simulink model "linear_flight_controller_payload"  (R2020a)
settings: Solver=FixedStepAuto  StartTime=0.0  StopTime=50  FixedStep=0.005  RelTol=1e-3
InitFcn:
  | flight_controller_payload_setup % Script to setup workspace
values from neighbouring files (symbols this model uses):
  C_Dx = 0.2    [PID_design_setup.m]    (also in flight_controller_payload_setup.m)
  C_Dz = 0.2    [PID_design_setup.m]    (also in flight_controller_payload_setup.m)
  C_px = 0.05    [flight_controller_payload_setup.m]
  C_pz = 0.05    [flight_controller_payload_setup.m]
  cbeta = 0.05    [flight_controller_payload_setup.m]
  dtheta_sp_max = 120*pi/180    (= 2.09439510239)    [flight_controller_payload_setup.m]
  dtheta_sp_min = -120*pi/180    (= -2.09439510239)    [flight_controller_payload_setup.m]
  dx_sp_max = 12    [flight_controller_payload_setup.m]
  dx_sp_min = -12    [flight_controller_payload_setup.m]
  dz_sp_max = 12    [flight_controller_payload_setup.m]
  dz_sp_min = -12    [flight_controller_payload_setup.m]
  g = -9.81    [PID_design_setup.m]    (also in flight_controller_payload_setup.m)
  I_yy = 0.235    [PID_design_setup.m]    (also in flight_controller_payload_setup.m)
  ki_dtheta = kp_dtheta*z_c    (= 0.1)    [PID_design_setup.m]
  kp_dtheta = 10^(K_dB/20)    [PID_design_setup.m]
  l = 1    [flight_controller_payload_setup.m]
  M = 4.5    [PID_design_setup.m]    (also in flight_controller_payload_setup.m)
  m = 2    [flight_controller_payload_setup.m]
  MM = [-1, 1 ... (first row only)    [flight_controller_payload_setup.m]    (also in flight_controller_setup.m = [-1/sqrt(2), -1)
  N_dtheta = Inf    (= inf)    [flight_controller_payload_setup.m]
  N_dx = 5*2*pi    (= 31.4159265359)    [flight_controller_payload_setup.m]
  N_dz = 5*2*pi    (= 31.4159265359)    [flight_controller_payload_setup.m]
  r = 0.49*1/sqrt(2)    [PID_design_setup.m]    (also in flight_controller_payload_setup.m)
  rho = 1.225    [PID_design_setup.m]    (also in flight_controller_payload_setup.m)
  sigma = 0    [flight_controller_payload_setup.m]
  tau = 0.07    [PID_design_setup.m]    (also in flight_controller_payload_setup.m)
  theta_sp_max = 30*pi/180    (= 0.523598775598)    [flight_controller_payload_setup.m]
  theta_sp_min = -30*pi/180    (= -0.523598775598)    [flight_controller_payload_setup.m]
  Ts_excite = 0    [flight_controller_payload_setup.m]
  Ts_mpc = 0.03    [flight_controller_payload_setup.m]
  u0 = -0.5*M*g*[1; 1]    [flight_controller_payload_setup.m]
  var_excite = 0    [flight_controller_payload_setup.m]
  x0 = zeros(nx,1)    [flight_controller_payload_setup.m]    (also in flight_controller_setup.m = zeros(6,1))
  x0_no_load = zeros(6,1)    [flight_controller_payload_setup.m]
undefined symbols (not defined in the file or in its folder): A_lin, B_lin, kd_dtheta, kd_dx, kd_dz, ki_dx, ki_dz, kp_dx, kp_dz, kp_theta, kp_x, kp_z
libraries: simulink x26, dspstat3 x8, mpclib x2
(part 2 of 3)

== system linear_flight_controller_payload/PID controllers WITHOUT payload/Angular rate controller1 ==
  note: PID to use auto tuning from simulink
  dtheta_sp : Inport
  X : Inport  Port=2
  Demux1 : Demux  Outputs=6
  Derivative : Derivative
  Gain : Gain  Gain=kd_dtheta
  I : Gain  Gain=ki_dtheta
  Integrator Limited : Integrator  LimitOutput=on  UpperSaturationLimit=10  LowerSaturationLimit=-10
  Low Pass Filter : TransferFcn  Denominator=[1/N_dtheta, 1]
  P : Gain  Gain=kp_dtheta
  PID Omega Controller : simulink/Continuous/PID Controller  Commented=on  Controller=PID  Form=Parallel  TimeDomain=Continuous-time  UseExternalTs=off  SampleTime=-1  IntegratorMethod=Forward Euler  FilterMethod=Forward Euler  ControllerParametersSource=internal  P=kp_dtheta  I=ki_dtheta  D=kd_dtheta  UseFilter=on  N=N_dtheta  TunerSelectOption=Transfer Function Based (PID Tuner App)  InitialConditionSource=internal  InitialConditionForIntegrator=0  InitialConditionForFilter=0  DifferentiatorICPrevScaledInput=0  ExternalReset=none  TrackingMode=off  Kt=1  LimitOutput=off  UpperSaturationLimit=inf  LowerSaturationLimit=-inf  LinearizeAsGain=on  AntiWindupMode=none  Kb=1  POutMin=[]  POutMax=[]  IOutMin=[]  IOutMax=[]  DOutMin=[]  DOutMax=[]  NOutMin=[]  NOutMax=[]  SumOutMin=[]  SumOutMax=[]  SaturationOutMin=[]  SaturationOutMax=[]  PParamMin=[]  PParamMax=[]  IParamMin=[]  IParamMax=[]  DParamMin=[]  DParamMax=[]  NParamMin=[]  NParamMax=[]  KbParamMin=[]  KbParamMax=[]  KtParamMin=[]  KtParamMax=[]  KbOutMin=[]  KbOutMax=[]  KtOutMin=[]  KtOutMax=[]  IntegratorOutMin=[]  IntegratorOutMax=[]  FilterOutMin=[]  FilterOutMax=[]  SumI1OutMin=[]  SumI1OutMax=[]  SumI2OutMin=[]  SumI2OutMax=[]  SumI3OutMin=[]  SumI3OutMax=[]  SumI4OutMin=[]  SumI4OutMax=[]  SumDOutMin=[]  SumDOutMax=[]  DifferentiatorOutMin=[]  DifferentiatorOutMax=[]  FilterDiffOutCoefMin=[]  FilterDiffOutCoefMax=[]  ReciprocalOutMin=[]  ReciprocalOutMax=[]  SumDenOutMin=[]  SumDenOutMax=[]  SumNumOutMin=[]  SumNumOutMax=[]  DivideOutMin=[]  DivideOutMax=[]  UdiffTsProdOutMin=[]  UdiffTsProdOutMax=[]  NTsProdOutMin=[]  NTsProdOutMax=[]  UintegralTsProdOutMin=[]  UintegralTsProdOutMax=[]  UngainTsProdOutMin=[]  UngainTsProdOutMax=[]  IntegratorContinuousStateAttributes=''  IntegratorStateMustResolveToSignalObject=off  IntegratorRTWStateStorageClass=Auto  FilterContinuousStateAttributes=''  FilterStateMustResolveToSignalObject=off  FilterRTWStateStorageClass=Auto  ParallelPVariant=InternalParameters  IdealPVariant=Disabled  IVariant=InternalParameters  DVariant=InternalParameters  IntegratorVariant=Continuous  SatVariant=Disabled  AWVariant=Passthrough  PCopyVariant=Disabled  TRVariant=Disabled  FdbkBlocksVariant=Forward  IdealPFdbkVariant=Disabled  SatFdbkVariant=Disabled  DerivativeFilterVariant=ContFilter  NVariant=InternalParameters  NCopyVariant=Disabled  FilterICVariant=InternalICsFilter  IntegratorICVariant=InternalICs  ExternalResetVariant=Disabled  TRSumVariant=Passthrough  SumFdbkVariant=Disabled  SumVariant=Sum_PID  TsampFilterVariant=InternalTs  TsampNgainVariant=Passthrough  TsampIntegralVariant=Passthrough
  Sum : Sum  Inputs=|+-
  Sum1 : Sum  Inputs=++-
  Sum2 : Sum  Inputs=++|
  delta_E : Outport
  wires:
  dtheta_sp/1 -> Sum/1
  Sum/1 -> P/1, Integrator Limited/1, PID Omega Controller/1
  Integrator Limited/1 -> I/1
  Derivative/1 -> Gain/1
  I/1 -> Sum1/2
  P/1 -> Sum1/1
  Gain/1 -> Sum1/3
  Sum1/1 -> Sum2/2
  Sum2/1 -> delta_E/1
  PID Omega Controller/1 -> Sum2/1
  Low Pass Filter/1 -> Derivative/1
  X/1 -> Demux1/1
  Demux1/6 -> Low Pass Filter/1, Sum/2  "dtheta"

== system linear_flight_controller_payload/PID controllers WITHOUT payload/Motor Mixing Algorithm1 ==
  delta_E : Inport
  delta_T : Inport  Port=2
  Mixing Matrix : Gain  Gain=MM  Multiplication=Matrix(K*u)
  Mux : Mux  Inputs=2
  Signal Specification : SignalSpecification  Dimensions=[2, 1]
  u : Outport  LockScale=on
  wires:
  delta_T/1 -> Mux/2
  delta_E/1 -> Mux/1
  Mixing Matrix/1 -> u/1
  Mux/1 -> Signal Specification/1
  Signal Specification/1 -> Mixing Matrix/1

== system linear_flight_controller_payload/PID controllers WITHOUT payload/Plant WITHOUT payload ==
  u : Inport  PortDimensions=[2, 1]
  Integrator : Integrator  InitialCondition=x0_no_load
  MATLAB Function1 : MATLAB Function  TreatAsAtomicUnit=on
  Motors : Subsystem
  Signal Specification : SignalSpecification  Dimensions=2
  parameters : Subsystem
  x : Outport
  wires:
  Motors/1(T) -> Signal Specification/1
  Signal Specification/1 -> MATLAB Function1/2(u)
  MATLAB Function1/1(dx) -> Integrator/1
  u/1 -> Motors/1(T_r)
  parameters/1(parameters) -> MATLAB Function1/3(params)
  Integrator/1 -> x/1, MATLAB Function1/1(x)

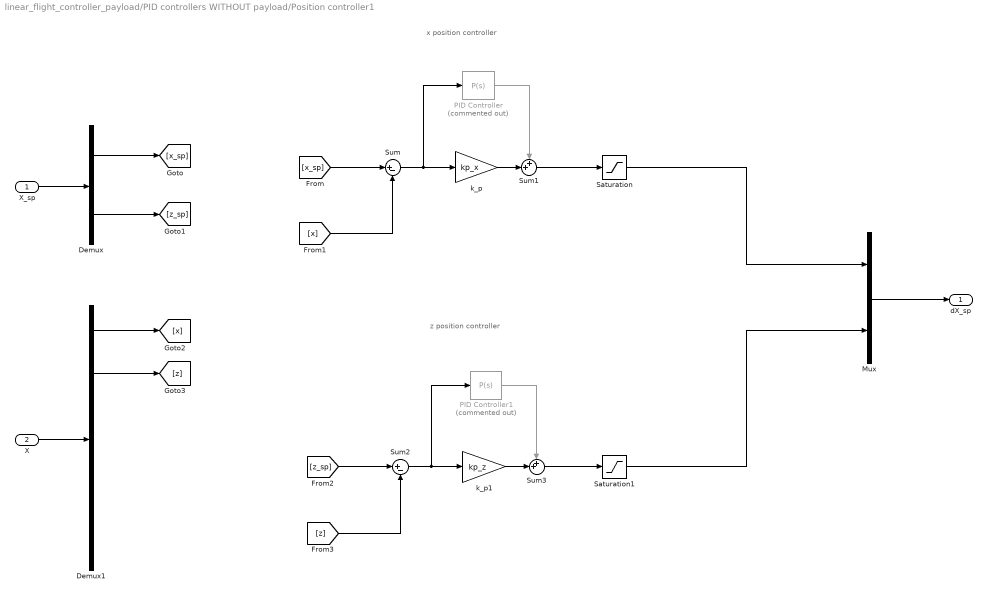
== system linear_flight_controller_payload/PID controllers WITHOUT payload/Position controller1 ==
  note: x position controller
  note: z position controller
  X_sp : Inport
  X : Inport  Port=2
  Demux : Demux  Outputs=2
  Demux1 : Demux  Outputs=6
  Mux : Mux  Inputs=2
  PID Controller : simulink/Continuous/PID Controller  Commented=on  Controller=P  Form=Parallel  TimeDomain=Continuous-time  UseExternalTs=off  SampleTime=-1  IntegratorMethod=Forward Euler  FilterMethod=Forward Euler  ControllerParametersSource=internal  P=20  I=1  D=0  UseFilter=on  N=100  TunerSelectOption=Transfer Function Based (PID Tuner App)  InitialConditionSource=internal  InitialConditionForIntegrator=0  InitialConditionForFilter=0  DifferentiatorICPrevScaledInput=0  ExternalReset=none  TrackingMode=off  Kt=1  LimitOutput=off  UpperSaturationLimit=inf  LowerSaturationLimit=-inf  LinearizeAsGain=on  AntiWindupMode=none  Kb=1  POutMin=[]  POutMax=[]  IOutMin=[]  IOutMax=[]  DOutMin=[]  DOutMax=[]  NOutMin=[]  NOutMax=[]  SumOutMin=[]  SumOutMax=[]  SaturationOutMin=[]  SaturationOutMax=[]  PParamMin=[]  PParamMax=[]  IParamMin=[]  IParamMax=[]  DParamMin=[]  DParamMax=[]  NParamMin=[]  NParamMax=[]  KbParamMin=[]  KbParamMax=[]  KtParamMin=[]  KtParamMax=[]  KbOutMin=[]  KbOutMax=[]  KtOutMin=[]  KtOutMax=[]  IntegratorOutMin=[]  IntegratorOutMax=[]  FilterOutMin=[]  FilterOutMax=[]  SumI1OutMin=[]  SumI1OutMax=[]  SumI2OutMin=[]  SumI2OutMax=[]  SumI3OutMin=[]  SumI3OutMax=[]  SumI4OutMin=[]  SumI4OutMax=[]  SumDOutMin=[]  SumDOutMax=[]  DifferentiatorOutMin=[]  DifferentiatorOutMax=[]  FilterDiffOutCoefMin=[]  FilterDiffOutCoefMax=[]  ReciprocalOutMin=[]  ReciprocalOutMax=[]  SumDenOutMin=[]  SumDenOutMax=[]  SumNumOutMin=[]  SumNumOutMax=[]  DivideOutMin=[]  DivideOutMax=[]  UdiffTsProdOutMin=[]  UdiffTsProdOutMax=[]  NTsProdOutMin=[]  NTsProdOutMax=[]  UintegralTsProdOutMin=[]  UintegralTsProdOutMax=[]  UngainTsProdOutMin=[]  UngainTsProdOutMax=[]  IntegratorContinuousStateAttributes=''  IntegratorStateMustResolveToSignalObject=off  IntegratorRTWStateStorageClass=Auto  FilterContinuousStateAttributes=''  FilterStateMustResolveToSignalObject=off  FilterRTWStateStorageClass=Auto  ParallelPVariant=InternalParameters  IdealPVariant=Disabled  IVariant=Disabled  DVariant=Disabled  IntegratorVariant=Disabled  SatVariant=Disabled  AWVariant=Disabled  PCopyVariant=Disabled  TRVariant=Disabled  FdbkBlocksVariant=Forward  IdealPFdbkVariant=Disabled  SatFdbkVariant=Disabled  DerivativeFilterVariant=Disabled  NVariant=Disabled  NCopyVariant=Disabled_SignalSpec  FilterICVariant=Disabled  IntegratorICVariant=Disabled  ExternalResetVariant=Disabled  TRSumVariant=Passthrough  SumFdbkVariant=Disabled  SumVariant=Passthrough_P  TsampFilterVariant=InternalTs  TsampNgainVariant=Passthrough  TsampIntegralVariant=Disabled_SignalSpec
  PID Controller1 : simulink/Continuous/PID Controller  Commented=on  Controller=P  Form=Parallel  TimeDomain=Continuous-time  UseExternalTs=off  SampleTime=-1  IntegratorMethod=Forward Euler  FilterMethod=Forward Euler  ControllerParametersSource=internal  P=1  I=1  D=0  UseFilter=on  N=100  TunerSelectOption=Transfer Function Based (PID Tuner App)  InitialConditionSource=internal  InitialConditionForIntegrator=0  InitialConditionForFilter=0  DifferentiatorICPrevScaledInput=0  ExternalReset=none  TrackingMode=off  Kt=1  LimitOutput=off  UpperSaturationLimit=inf  LowerSaturationLimit=-inf  LinearizeAsGain=on  AntiWindupMode=none  Kb=1  POutMin=[]  POutMax=[]  IOutMin=[]  IOutMax=[]  DOutMin=[]  DOutMax=[]  NOutMin=[]  NOutMax=[]  SumOutMin=[]  SumOutMax=[]  SaturationOutMin=[]  SaturationOutMax=[]  PParamMin=[]  PParamMax=[]  IParamMin=[]  IParamMax=[]  DParamMin=[]  DParamMax=[]  NParamMin=[]  NParamMax=[]  KbParamMin=[]  KbParamMax=[]  KtParamMin=[]  KtParamMax=[]  KbOutMin=[]  KbOutMax=[]  KtOutMin=[]  KtOutMax=[]  IntegratorOutMin=[]  IntegratorOutMax=[]  FilterOutMin=[]  FilterOutMax=[]  SumI1OutMin=[]  SumI1OutMax=[]  SumI2OutMin=[]  SumI2OutMax=[]  SumI3OutMin=[]  SumI3OutMax=[]  SumI4OutMin=[]  SumI4OutMax=[]  SumDOutMin=[]  SumDOutMax=[]  DifferentiatorOutMin=[]  DifferentiatorOutMax=[]  FilterDiffOutCoefMin=[]  FilterDiffOutCoefMax=[]  ReciprocalOutMin=[]  ReciprocalOutMax=[]  SumDenOutMin=[]  SumDenOutMax=[]  SumNumOutMin=[]  SumNumOutMax=[]  DivideOutMin=[]  DivideOutMax=[]  UdiffTsProdOutMin=[]  UdiffTsProdOutMax=[]  NTsProdOutMin=[]  NTsProdOutMax=[]  UintegralTsProdOutMin=[]  UintegralTsProdOutMax=[]  UngainTsProdOutMin=[]  UngainTsProdOutMax=[]  IntegratorContinuousStateAttributes=''  IntegratorStateMustResolveToSignalObject=off  IntegratorRTWStateStorageClass=Auto  FilterContinuousStateAttributes=''  FilterStateMustResolveToSignalObject=off  FilterRTWStateStorageClass=Auto  ParallelPVariant=InternalParameters  IdealPVariant=Disabled  IVariant=Disabled  DVariant=Disabled  IntegratorVariant=Disabled  SatVariant=Disabled  AWVariant=Disabled  PCopyVariant=Disabled  TRVariant=Disabled  FdbkBlocksVariant=Forward  IdealPFdbkVariant=Disabled  SatFdbkVariant=Disabled  DerivativeFilterVariant=Disabled  NVariant=Disabled  NCopyVariant=Disabled_SignalSpec  FilterICVariant=Disabled  IntegratorICVariant=Disabled  ExternalResetVariant=Disabled  TRSumVariant=Passthrough  SumFdbkVariant=Disabled  SumVariant=Passthrough_P  TsampFilterVariant=InternalTs  TsampNgainVariant=Passthrough  TsampIntegralVariant=Disabled_SignalSpec
  Saturation : Saturate  UpperLimit=dx_sp_max  LowerLimit=dx_sp_min
  Saturation1 : Saturate  UpperLimit=dz_sp_max  LowerLimit=dz_sp_min
  Sum : Sum  Inputs=|+-
  Sum1 : Sum  Inputs=++|
  Sum2 : Sum  Inputs=|+-
  Sum3 : Sum  Inputs=++|
  k_p : Gain  Gain=kp_x
  k_p1 : Gain  Gain=kp_z
  dX_sp : Outport
  wires:
  Sum/1 -> PID Controller/1, k_p/1
  k_p/1 -> Sum1/2
  PID Controller/1 -> Sum1/1
  X_sp/1 -> Demux/1
  Demux/2 -> [z_sp]
  Demux/1 -> [x_sp]
  X/1 -> Demux1/1
  Demux1/1 -> [x]
  Demux1/2 -> [z]
  [x_sp] -> Sum/1
  [x] -> Sum/2
  Sum2/1 -> PID Controller1/1, k_p1/1
  [z] -> Sum2/2
  [z_sp] -> Sum2/1
  PID Controller1/1 -> Sum3/1
  k_p1/1 -> Sum3/2
  Mux/1 -> dX_sp/1
  Sum1/1 -> Saturation/1
  Sum3/1 -> Saturation1/1
  Saturation1/1 -> Mux/2
  Saturation/1 -> Mux/1

== system linear_flight_controller_payload/PID controllers WITHOUT payload/Subsystem1 ==
  X : Inport
  Demux : Demux  Outputs=6
  theta : Outport
  wires:
  X/1 -> Demux/1
  Demux/3 -> theta/1

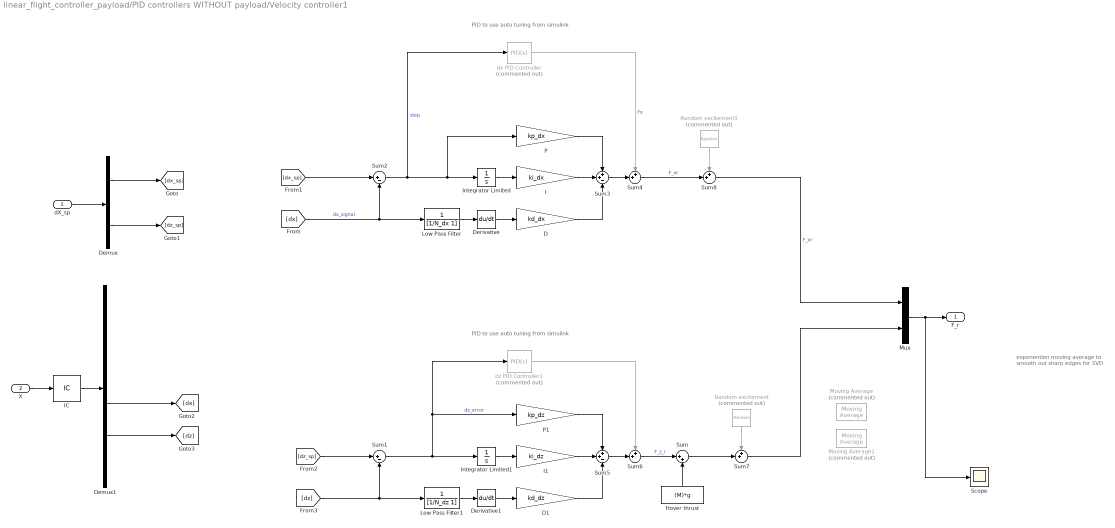
== system linear_flight_controller_payload/PID controllers WITHOUT payload/Velocity controller1 ==
  note: exponention moving average
      | to smooth out sharp edges for SVD
  note: PID to use auto tuning from simulink
  note: PID to use auto tuning from simulink
  dX_sp : Inport
  X : Inport  Port=2
  D : Gain  Gain=kd_dx
  D1 : Gain  Gain=kd_dz
  Demux : Demux  Outputs=2
  Demux1 : Demux  Outputs=6
  Derivative : Derivative
  Derivative1 : Derivative
  Hover thrust : Constant  Value=(M)*g
  I : Gain  Gain=ki_dx
  I1 : Gain  Gain=ki_dz
  IC : InitialCondition  Value=x0_no_load
  Integrator Limited : Integrator  LimitOutput=on  UpperSaturationLimit=10  LowerSaturationLimit=-10
  Integrator Limited1 : Integrator  LimitOutput=on  UpperSaturationLimit=10  LowerSaturationLimit=-10
  Low Pass Filter : TransferFcn  Denominator=[1/N_dx 1]
  Low Pass Filter1 : TransferFcn  Denominator=[1/N_dz 1]
  Moving Average : dspstat3/Moving Average  Commented=on  Method=Exponential weighting  ForgettingFactorPort=off  SpecifyWindowLength=on  WindowLength=4  ForgettingFactor=lambda  SimulateUsing=Code generation
  Moving Average1 : dspstat3/Moving Average  Commented=on  Method=Exponential weighting  ForgettingFactorPort=off  SpecifyWindowLength=on  WindowLength=4  ForgettingFactor=lambda  SimulateUsing=Code generation
  Mux : Mux  Inputs=2
  P : Gain  Gain=kp_dx
  P1 : Gain  Gain=kp_dz
  Random excitement : RandomNumber  Commented=on  Variance=var_excite  SampleTime=Ts_excite
  Random excitement1 : RandomNumber  Commented=on  Variance=var_excite  Seed=1  SampleTime=Ts_excite
  Scope : Scope
  Sum : Sum  Inputs=|++
  Sum1 : Sum  Inputs=|+-
  Sum2 : Sum  Inputs=|+-
  Sum3 : Sum  Inputs=++-
  Sum{4,6..8} (4 alike) : Sum  Inputs=++|
  Sum5 : Sum  Inputs=++-
  dx PID Controller : simulink/Continuous/PID Controller  Commented=on  Controller=PID  Form=Parallel  TimeDomain=Continuous-time  UseExternalTs=off  SampleTime=-1  IntegratorMethod=Forward Euler  FilterMethod=Forward Euler  ControllerParametersSource=internal  P=kp_dx  I=ki_dx  D=kd_dx  UseFilter=on  N=N_dx  TunerSelectOption=Transfer Function Based (PID Tuner App)  InitialConditionSource=internal  InitialConditionForIntegrator=0  InitialConditionForFilter=0  DifferentiatorICPrevScaledInput=0  ExternalReset=none  TrackingMode=off  Kt=1  LimitOutput=off  UpperSaturationLimit=inf  LowerSaturationLimit=-inf  LinearizeAsGain=on  AntiWindupMode=none  Kb=1  POutMin=[]  POutMax=[]  IOutMin=[]  IOutMax=[]  DOutMin=[]  DOutMax=[]  NOutMin=[]  NOutMax=[]  SumOutMin=[]  SumOutMax=[]  SaturationOutMin=[]  SaturationOutMax=[]  PParamMin=[]  PParamMax=[]  IParamMin=[]  IParamMax=[]  DParamMin=[]  DParamMax=[]  NParamMin=[]  NParamMax=[]  KbParamMin=[]  KbParamMax=[]  KtParamMin=[]  KtParamMax=[]  KbOutMin=[]  KbOutMax=[]  KtOutMin=[]  KtOutMax=[]  IntegratorOutMin=[]  IntegratorOutMax=[]  FilterOutMin=[]  FilterOutMax=[]  SumI1OutMin=[]  SumI1OutMax=[]  SumI2OutMin=[]  SumI2OutMax=[]  SumI3OutMin=[]  SumI3OutMax=[]  SumI4OutMin=[]  SumI4OutMax=[]  SumDOutMin=[]  SumDOutMax=[]  DifferentiatorOutMin=[]  DifferentiatorOutMax=[]  FilterDiffOutCoefMin=[]  FilterDiffOutCoefMax=[]  ReciprocalOutMin=[]  ReciprocalOutMax=[]  SumDenOutMin=[]  SumDenOutMax=[]  SumNumOutMin=[]  SumNumOutMax=[]  DivideOutMin=[]  DivideOutMax=[]  UdiffTsProdOutMin=[]  UdiffTsProdOutMax=[]  NTsProdOutMin=[]  NTsProdOutMax=[]  UintegralTsProdOutMin=[]  UintegralTsProdOutMax=[]  UngainTsProdOutMin=[]  UngainTsProdOutMax=[]  IntegratorContinuousStateAttributes=''  IntegratorStateMustResolveToSignalObject=off  IntegratorRTWStateStorageClass=Auto  FilterContinuousStateAttributes=''  FilterStateMustResolveToSignalObject=off  FilterRTWStateStorageClass=Auto  ParallelPVariant=InternalParameters  IdealPVariant=Disabled  IVariant=InternalParameters  DVariant=InternalParameters  IntegratorVariant=Continuous  SatVariant=Disabled  AWVariant=Passthrough  PCopyVariant=Disabled  TRVariant=Disabled  FdbkBlocksVariant=Forward  IdealPFdbkVariant=Disabled  SatFdbkVariant=Disabled  DerivativeFilterVariant=ContFilter  NVariant=InternalParameters  NCopyVariant=Disabled  FilterICVariant=InternalICsFilter  IntegratorICVariant=InternalICs  ExternalResetVariant=Disabled  TRSumVariant=Passthrough  SumFdbkVariant=Disabled  SumVariant=Sum_PID  TsampFilterVariant=InternalTs  TsampNgainVariant=Passthrough  TsampIntegralVariant=Passthrough
  dz PID Controller1 : simulink/Continuous/PID Controller  Commented=on  Controller=PID  Form=Parallel  TimeDomain=Continuous-time  UseExternalTs=off  SampleTime=-1  IntegratorMethod=Forward Euler  FilterMethod=Forward Euler  ControllerParametersSource=internal  P=kp_dz  I=ki_dz  D=kd_dz  UseFilter=on  N=N_dz  TunerSelectOption=Transfer Function Based (PID Tuner App)  InitialConditionSource=internal  InitialConditionForIntegrator=0  InitialConditionForFilter=0  DifferentiatorICPrevScaledInput=0  ExternalReset=none  TrackingMode=off  Kt=1  LimitOutput=off  UpperSaturationLimit=inf  LowerSaturationLimit=-inf  LinearizeAsGain=on  AntiWindupMode=none  Kb=1  POutMin=[]  POutMax=[]  IOutMin=[]  IOutMax=[]  DOutMin=[]  DOutMax=[]  NOutMin=[]  NOutMax=[]  SumOutMin=[]  SumOutMax=[]  SaturationOutMin=[]  SaturationOutMax=[]  PParamMin=[]  PParamMax=[]  IParamMin=[]  IParamMax=[]  DParamMin=[]  DParamMax=[]  NParamMin=[]  NParamMax=[]  KbParamMin=[]  KbParamMax=[]  KtParamMin=[]  KtParamMax=[]  KbOutMin=[]  KbOutMax=[]  KtOutMin=[]  KtOutMax=[]  IntegratorOutMin=[]  IntegratorOutMax=[]  FilterOutMin=[]  FilterOutMax=[]  SumI1OutMin=[]  SumI1OutMax=[]  SumI2OutMin=[]  SumI2OutMax=[]  SumI3OutMin=[]  SumI3OutMax=[]  SumI4OutMin=[]  SumI4OutMax=[]  SumDOutMin=[]  SumDOutMax=[]  DifferentiatorOutMin=[]  DifferentiatorOutMax=[]  FilterDiffOutCoefMin=[]  FilterDiffOutCoefMax=[]  ReciprocalOutMin=[]  ReciprocalOutMax=[]  SumDenOutMin=[]  SumDenOutMax=[]  SumNumOutMin=[]  SumNumOutMax=[]  DivideOutMin=[]  DivideOutMax=[]  UdiffTsProdOutMin=[]  UdiffTsProdOutMax=[]  NTsProdOutMin=[]  NTsProdOutMax=[]  UintegralTsProdOutMin=[]  UintegralTsProdOutMax=[]  UngainTsProdOutMin=[]  UngainTsProdOutMax=[]  IntegratorContinuousStateAttributes=''  IntegratorStateMustResolveToSignalObject=off  IntegratorRTWStateStorageClass=Auto  FilterContinuousStateAttributes=''  FilterStateMustResolveToSignalObject=off  FilterRTWStateStorageClass=Auto  ParallelPVariant=InternalParameters  IdealPVariant=Disabled  IVariant=InternalParameters  DVariant=InternalParameters  IntegratorVariant=Continuous  SatVariant=Disabled  AWVariant=Passthrough  PCopyVariant=Disabled  TRVariant=Disabled  FdbkBlocksVariant=Forward  IdealPFdbkVariant=Disabled  SatFdbkVariant=Disabled  DerivativeFilterVariant=ContFilter  NVariant=InternalParameters  NCopyVariant=Disabled  FilterICVariant=InternalICsFilter  IntegratorICVariant=InternalICs  ExternalResetVariant=Disabled  TRSumVariant=Passthrough  SumFdbkVariant=Disabled  SumVariant=Sum_PID  TsampFilterVariant=InternalTs  TsampNgainVariant=Passthrough  TsampIntegralVariant=Passthrough
  F_r : Outport
  wires:
  Derivative/1 -> D/1
  Sum3/1 -> Sum4/2
  Sum2/1 -> dx PID Controller/1, P/1, Integrator Limited/1  "step"
  I/1 -> Sum3/2
  Integrator Limited/1 -> I/1
  dx PID Controller/1 -> Sum4/1  "Fx"
  P/1 -> Sum3/1
  Low Pass Filter/1 -> Derivative/1
  D/1 -> Sum3/3
  P1/1 -> Sum5/1
  Integrator Limited1/1 -> I1/1
  dz PID Controller1/1 -> Sum6/1
  I1/1 -> Sum5/2
  Sum1/1 -> P1/1, dz PID Controller1/1, Integrator Limited1/1  "dz_error"
  Sum5/1 -> Sum6/2
  Low Pass Filter1/1 -> Derivative1/1
  Derivative1/1 -> D1/1
  D1/1 -> Sum5/3
  dX_sp/1 -> Demux/1
  [dx] -> Sum2/2, Low Pass Filter/1  "dx_signal"
  [dx_sp] -> Sum2/1
  Demux/1 -> [dx_sp]
  Demux/2 -> [dz_sp]
  [dz] -> Sum1/2, Low Pass Filter1/1
  [dz_sp] -> Sum1/1
  Demux1/4 -> [dx]
  Demux1/5 -> [dz]
  Sum6/1 -> Sum/1  "F_z_r"
  Hover thrust/1 -> Sum/2
  IC/1 -> Demux1/1
  X/1 -> IC/1
  Sum8/1 -> Mux/1  "F_xr"
  Sum7/1 -> Mux/2
  Mux/1 -> Scope/1, F_r/1
  Random excitement/1 -> Sum7/1
  Sum/1 -> Sum7/2
  Random excitement1/1 -> Sum8/1
  Sum4/1 -> Sum8/2  "F_xr"

== system linear_flight_controller_payload/PID controllers and Plant/Angle controller1 ==
  theta_sp : Inport
  X : Inport  Port=2
  Demux1 : Demux  Outputs=nx
  Gain : Gain  Gain=kp_theta
  PID Controller : simulink/Continuous/PID Controller  Commented=on  Controller=P  Form=Parallel  TimeDomain=Continuous-time  UseExternalTs=off  SampleTime=-1  IntegratorMethod=Forward Euler  FilterMethod=Forward Euler  ControllerParametersSource=internal  P=kp_theta  I=1  D=0  UseFilter=on  N=100  TunerSelectOption=Transfer Function Based (PID Tuner App)  InitialConditionSource=internal  InitialConditionForIntegrator=0  InitialConditionForFilter=0  DifferentiatorICPrevScaledInput=0  ExternalReset=none  TrackingMode=off  Kt=1  LimitOutput=off  UpperSaturationLimit=inf  LowerSaturationLimit=-inf  LinearizeAsGain=on  AntiWindupMode=none  Kb=1  POutMin=[]  POutMax=[]  IOutMin=[]  IOutMax=[]  DOutMin=[]  DOutMax=[]  NOutMin=[]  NOutMax=[]  SumOutMin=[]  SumOutMax=[]  SaturationOutMin=[]  SaturationOutMax=[]  PParamMin=[]  PParamMax=[]  IParamMin=[]  IParamMax=[]  DParamMin=[]  DParamMax=[]  NParamMin=[]  NParamMax=[]  KbParamMin=[]  KbParamMax=[]  KtParamMin=[]  KtParamMax=[]  KbOutMin=[]  KbOutMax=[]  KtOutMin=[]  KtOutMax=[]  IntegratorOutMin=[]  IntegratorOutMax=[]  FilterOutMin=[]  FilterOutMax=[]  SumI1OutMin=[]  SumI1OutMax=[]  SumI2OutMin=[]  SumI2OutMax=[]  SumI3OutMin=[]  SumI3OutMax=[]  SumI4OutMin=[]  SumI4OutMax=[]  SumDOutMin=[]  SumDOutMax=[]  DifferentiatorOutMin=[]  DifferentiatorOutMax=[]  FilterDiffOutCoefMin=[]  FilterDiffOutCoefMax=[]  ReciprocalOutMin=[]  ReciprocalOutMax=[]  SumDenOutMin=[]  SumDenOutMax=[]  SumNumOutMin=[]  SumNumOutMax=[]  DivideOutMin=[]  DivideOutMax=[]  UdiffTsProdOutMin=[]  UdiffTsProdOutMax=[]  NTsProdOutMin=[]  NTsProdOutMax=[]  UintegralTsProdOutMin=[]  UintegralTsProdOutMax=[]  UngainTsProdOutMin=[]  UngainTsProdOutMax=[]  IntegratorContinuousStateAttributes=''  IntegratorStateMustResolveToSignalObject=off  IntegratorRTWStateStorageClass=Auto  FilterContinuousStateAttributes=''  FilterStateMustResolveToSignalObject=off  FilterRTWStateStorageClass=Auto  ParallelPVariant=InternalParameters  IdealPVariant=Disabled  IVariant=Disabled  DVariant=Disabled  IntegratorVariant=Disabled  SatVariant=Disabled  AWVariant=Disabled  PCopyVariant=Disabled  TRVariant=Disabled  FdbkBlocksVariant=Forward  IdealPFdbkVariant=Disabled  SatFdbkVariant=Disabled  DerivativeFilterVariant=Disabled  NVariant=Disabled  NCopyVariant=Disabled_SignalSpec  FilterICVariant=Disabled  IntegratorICVariant=Disabled  ExternalResetVariant=Disabled  TRSumVariant=Passthrough  SumFdbkVariant=Disabled  SumVariant=Passthrough_P  TsampFilterVariant=InternalTs  TsampNgainVariant=Passthrough  TsampIntegralVariant=Disabled_SignalSpec
  Sum : Sum  Inputs=++|
  Sum1 : Sum  Inputs=|+-
  limit : Saturate  UpperLimit=dtheta_sp_max  LowerLimit=dtheta_sp_min
  dtheta_sp : Outport
  wires:
  Sum1/1 -> PID Controller/1, Gain/1  "theta_error"
  theta_sp/1 -> Sum1/1
  PID Controller/1 -> Sum/1
  Gain/1 -> Sum/2
  X/1 -> Demux1/1
  Demux1/3 -> Sum1/2
  Sum/1 -> limit/1
  limit/1 -> dtheta_sp/1

== system linear_flight_controller_payload/PID controllers and Plant/Angular rate controller1 ==
  note: PID to use auto tuning from simulink
  dtheta_sp : Inport
  X : Inport  Port=2
  Demux1 : Demux  Outputs=nx
  Derivative : Derivative
  Gain : Gain  Gain=kd_dtheta
  I : Gain  Gain=ki_dtheta
  Integrator Limited : Integrator  LimitOutput=on  UpperSaturationLimit=10  LowerSaturationLimit=-10
  Low Pass Filter : TransferFcn  Denominator=[1/N_dtheta, 1]
  P : Gain  Gain=kp_dtheta
  PID Omega Controller : simulink/Continuous/PID Controller  Commented=on  Controller=PID  Form=Parallel  TimeDomain=Continuous-time  UseExternalTs=off  SampleTime=-1  IntegratorMethod=Forward Euler  FilterMethod=Forward Euler  ControllerParametersSource=internal  P=kp_dtheta  I=ki_dtheta  D=kd_dtheta  UseFilter=on  N=N_dtheta  TunerSelectOption=Transfer Function Based (PID Tuner App)  InitialConditionSource=internal  InitialConditionForIntegrator=0  InitialConditionForFilter=0  DifferentiatorICPrevScaledInput=0  ExternalReset=none  TrackingMode=off  Kt=1  LimitOutput=off  UpperSaturationLimit=inf  LowerSaturationLimit=-inf  LinearizeAsGain=on  AntiWindupMode=none  Kb=1  POutMin=[]  POutMax=[]  IOutMin=[]  IOutMax=[]  DOutMin=[]  DOutMax=[]  NOutMin=[]  NOutMax=[]  SumOutMin=[]  SumOutMax=[]  SaturationOutMin=[]  SaturationOutMax=[]  PParamMin=[]  PParamMax=[]  IParamMin=[]  IParamMax=[]  DParamMin=[]  DParamMax=[]  NParamMin=[]  NParamMax=[]  KbParamMin=[]  KbParamMax=[]  KtParamMin=[]  KtParamMax=[]  KbOutMin=[]  KbOutMax=[]  KtOutMin=[]  KtOutMax=[]  IntegratorOutMin=[]  IntegratorOutMax=[]  FilterOutMin=[]  FilterOutMax=[]  SumI1OutMin=[]  SumI1OutMax=[]  SumI2OutMin=[]  SumI2OutMax=[]  SumI3OutMin=[]  SumI3OutMax=[]  SumI4OutMin=[]  SumI4OutMax=[]  SumDOutMin=[]  SumDOutMax=[]  DifferentiatorOutMin=[]  DifferentiatorOutMax=[]  FilterDiffOutCoefMin=[]  FilterDiffOutCoefMax=[]  ReciprocalOutMin=[]  ReciprocalOutMax=[]  SumDenOutMin=[]  SumDenOutMax=[]  SumNumOutMin=[]  SumNumOutMax=[]  DivideOutMin=[]  DivideOutMax=[]  UdiffTsProdOutMin=[]  UdiffTsProdOutMax=[]  NTsProdOutMin=[]  NTsProdOutMax=[]  UintegralTsProdOutMin=[]  UintegralTsProdOutMax=[]  UngainTsProdOutMin=[]  UngainTsProdOutMax=[]  IntegratorContinuousStateAttributes=''  IntegratorStateMustResolveToSignalObject=off  IntegratorRTWStateStorageClass=Auto  FilterContinuousStateAttributes=''  FilterStateMustResolveToSignalObject=off  FilterRTWStateStorageClass=Auto  ParallelPVariant=InternalParameters  IdealPVariant=Disabled  IVariant=InternalParameters  DVariant=InternalParameters  IntegratorVariant=Continuous  SatVariant=Disabled  AWVariant=Passthrough  PCopyVariant=Disabled  TRVariant=Disabled  FdbkBlocksVariant=Forward  IdealPFdbkVariant=Disabled  SatFdbkVariant=Disabled  DerivativeFilterVariant=ContFilter  NVariant=InternalParameters  NCopyVariant=Disabled  FilterICVariant=InternalICsFilter  IntegratorICVariant=InternalICs  ExternalResetVariant=Disabled  TRSumVariant=Passthrough  SumFdbkVariant=Disabled  SumVariant=Sum_PID  TsampFilterVariant=InternalTs  TsampNgainVariant=Passthrough  TsampIntegralVariant=Passthrough
  Sum : Sum  Inputs=|+-
  Sum1 : Sum  Inputs=++-
  Sum2 : Sum  Inputs=++|
  delta_E : Outport
  wires:
  dtheta_sp/1 -> Sum/1
  Sum/1 -> P/1, Integrator Limited/1, PID Omega Controller/1
  Integrator Limited/1 -> I/1
  Derivative/1 -> Gain/1
  I/1 -> Sum1/2
  P/1 -> Sum1/1
  Gain/1 -> Sum1/3
  Sum1/1 -> Sum2/2
  Sum2/1 -> delta_E/1
  PID Omega Controller/1 -> Sum2/1
  Low Pass Filter/1 -> Derivative/1
  X/1 -> Demux1/1
  Demux1/7 -> Low Pass Filter/1, Sum/2  "dtheta"

== system linear_flight_controller_payload/PID controllers and Plant/Motor Mixing Algorithm1 ==
  delta_E : Inport
  delta_T : Inport  Port=2
  Mixing Matrix : Gain  Gain=MM  Multiplication=Matrix(K*u)
  Mux : Mux  Inputs=2
  Signal Specification : SignalSpecification  Dimensions=[2, 1]
  u : Outport  LockScale=on
  wires:
  delta_T/1 -> Mux/2
  delta_E/1 -> Mux/1
  Mixing Matrix/1 -> u/1
  Mux/1 -> Signal Specification/1
  Signal Specification/1 -> Mixing Matrix/1

== system linear_flight_controller_payload/PID controllers and Plant/Plant1 ==
  u : Inport  PortDimensions=[2, 1]
  Integrator : Integrator  InitialCondition=x0
  MATLAB Function1 : MATLAB Function  TreatAsAtomicUnit=on
  Motors : Subsystem
  Signal Specification : SignalSpecification  Dimensions=2
  parameters : Subsystem
  x : Outport
  wires:
  Motors/1(T) -> Signal Specification/1
  Signal Specification/1 -> MATLAB Function1/2(u)
  MATLAB Function1/1(dx) -> Integrator/1
  u/1 -> Motors/1(T_r)
  parameters/1(parameters) -> MATLAB Function1/3(params)
  Integrator/1 -> x/1, MATLAB Function1/1(x)

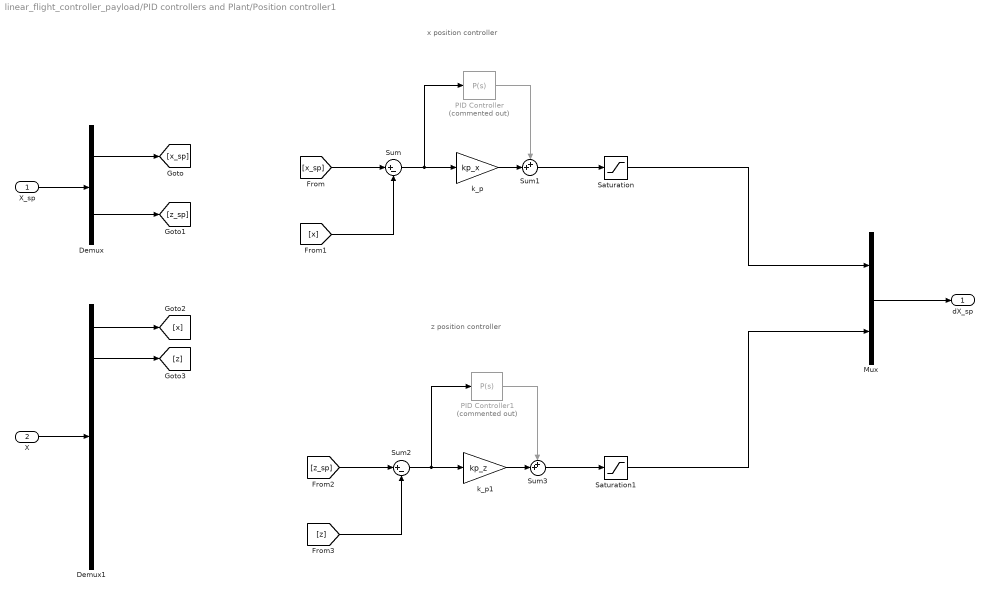
== system linear_flight_controller_payload/PID controllers and Plant/Position controller1 ==
  note: x position controller
  note: z position controller
  X_sp : Inport
  X : Inport  Port=2
  Demux : Demux  Outputs=2
  Demux1 : Demux  Outputs=nx
  Mux : Mux  Inputs=2
  PID Controller : simulink/Continuous/PID Controller  Commented=on  Controller=P  Form=Parallel  TimeDomain=Continuous-time  UseExternalTs=off  SampleTime=-1  IntegratorMethod=Forward Euler  FilterMethod=Forward Euler  ControllerParametersSource=internal  P=20  I=1  D=0  UseFilter=on  N=100  TunerSelectOption=Transfer Function Based (PID Tuner App)  InitialConditionSource=internal  InitialConditionForIntegrator=0  InitialConditionForFilter=0  DifferentiatorICPrevScaledInput=0  ExternalReset=none  TrackingMode=off  Kt=1  LimitOutput=off  UpperSaturationLimit=inf  LowerSaturationLimit=-inf  LinearizeAsGain=on  AntiWindupMode=none  Kb=1  POutMin=[]  POutMax=[]  IOutMin=[]  IOutMax=[]  DOutMin=[]  DOutMax=[]  NOutMin=[]  NOutMax=[]  SumOutMin=[]  SumOutMax=[]  SaturationOutMin=[]  SaturationOutMax=[]  PParamMin=[]  PParamMax=[]  IParamMin=[]  IParamMax=[]  DParamMin=[]  DParamMax=[]  NParamMin=[]  NParamMax=[]  KbParamMin=[]  KbParamMax=[]  KtParamMin=[]  KtParamMax=[]  KbOutMin=[]  KbOutMax=[]  KtOutMin=[]  KtOutMax=[]  IntegratorOutMin=[]  IntegratorOutMax=[]  FilterOutMin=[]  FilterOutMax=[]  SumI1OutMin=[]  SumI1OutMax=[]  SumI2OutMin=[]  SumI2OutMax=[]  SumI3OutMin=[]  SumI3OutMax=[]  SumI4OutMin=[]  SumI4OutMax=[]  SumDOutMin=[]  SumDOutMax=[]  DifferentiatorOutMin=[]  DifferentiatorOutMax=[]  FilterDiffOutCoefMin=[]  FilterDiffOutCoefMax=[]  ReciprocalOutMin=[]  ReciprocalOutMax=[]  SumDenOutMin=[]  SumDenOutMax=[]  SumNumOutMin=[]  SumNumOutMax=[]  DivideOutMin=[]  DivideOutMax=[]  UdiffTsProdOutMin=[]  UdiffTsProdOutMax=[]  NTsProdOutMin=[]  NTsProdOutMax=[]  UintegralTsProdOutMin=[]  UintegralTsProdOutMax=[]  UngainTsProdOutMin=[]  UngainTsProdOutMax=[]  IntegratorContinuousStateAttributes=''  IntegratorStateMustResolveToSignalObject=off  IntegratorRTWStateStorageClass=Auto  FilterContinuousStateAttributes=''  FilterStateMustResolveToSignalObject=off  FilterRTWStateStorageClass=Auto  ParallelPVariant=InternalParameters  IdealPVariant=Disabled  IVariant=Disabled  DVariant=Disabled  IntegratorVariant=Disabled  SatVariant=Disabled  AWVariant=Disabled  PCopyVariant=Disabled  TRVariant=Disabled  FdbkBlocksVariant=Forward  IdealPFdbkVariant=Disabled  SatFdbkVariant=Disabled  DerivativeFilterVariant=Disabled  NVariant=Disabled  NCopyVariant=Disabled_SignalSpec  FilterICVariant=Disabled  IntegratorICVariant=Disabled  ExternalResetVariant=Disabled  TRSumVariant=Passthrough  SumFdbkVariant=Disabled  SumVariant=Passthrough_P  TsampFilterVariant=InternalTs  TsampNgainVariant=Passthrough  TsampIntegralVariant=Disabled_SignalSpec
  PID Controller1 : simulink/Continuous/PID Controller  Commented=on  Controller=P  Form=Parallel  TimeDomain=Continuous-time  UseExternalTs=off  SampleTime=-1  IntegratorMethod=Forward Euler  FilterMethod=Forward Euler  ControllerParametersSource=internal  P=1  I=1  D=0  UseFilter=on  N=100  TunerSelectOption=Transfer Function Based (PID Tuner App)  InitialConditionSource=internal  InitialConditionForIntegrator=0  InitialConditionForFilter=0  DifferentiatorICPrevScaledInput=0  ExternalReset=none  TrackingMode=off  Kt=1  LimitOutput=off  UpperSaturationLimit=inf  LowerSaturationLimit=-inf  LinearizeAsGain=on  AntiWindupMode=none  Kb=1  POutMin=[]  POutMax=[]  IOutMin=[]  IOutMax=[]  DOutMin=[]  DOutMax=[]  NOutMin=[]  NOutMax=[]  SumOutMin=[]  SumOutMax=[]  SaturationOutMin=[]  SaturationOutMax=[]  PParamMin=[]  PParamMax=[]  IParamMin=[]  IParamMax=[]  DParamMin=[]  DParamMax=[]  NParamMin=[]  NParamMax=[]  KbParamMin=[]  KbParamMax=[]  KtParamMin=[]  KtParamMax=[]  KbOutMin=[]  KbOutMax=[]  KtOutMin=[]  KtOutMax=[]  IntegratorOutMin=[]  IntegratorOutMax=[]  FilterOutMin=[]  FilterOutMax=[]  SumI1OutMin=[]  SumI1OutMax=[]  SumI2OutMin=[]  SumI2OutMax=[]  SumI3OutMin=[]  SumI3OutMax=[]  SumI4OutMin=[]  SumI4OutMax=[]  SumDOutMin=[]  SumDOutMax=[]  DifferentiatorOutMin=[]  DifferentiatorOutMax=[]  FilterDiffOutCoefMin=[]  FilterDiffOutCoefMax=[]  ReciprocalOutMin=[]  ReciprocalOutMax=[]  SumDenOutMin=[]  SumDenOutMax=[]  SumNumOutMin=[]  SumNumOutMax=[]  DivideOutMin=[]  DivideOutMax=[]  UdiffTsProdOutMin=[]  UdiffTsProdOutMax=[]  NTsProdOutMin=[]  NTsProdOutMax=[]  UintegralTsProdOutMin=[]  UintegralTsProdOutMax=[]  UngainTsProdOutMin=[]  UngainTsProdOutMax=[]  IntegratorContinuousStateAttributes=''  IntegratorStateMustResolveToSignalObject=off  IntegratorRTWStateStorageClass=Auto  FilterContinuousStateAttributes=''  FilterStateMustResolveToSignalObject=off  FilterRTWStateStorageClass=Auto  ParallelPVariant=InternalParameters  IdealPVariant=Disabled  IVariant=Disabled  DVariant=Disabled  IntegratorVariant=Disabled  SatVariant=Disabled  AWVariant=Disabled  PCopyVariant=Disabled  TRVariant=Disabled  FdbkBlocksVariant=Forward  IdealPFdbkVariant=Disabled  SatFdbkVariant=Disabled  DerivativeFilterVariant=Disabled  NVariant=Disabled  NCopyVariant=Disabled_SignalSpec  FilterICVariant=Disabled  IntegratorICVariant=Disabled  ExternalResetVariant=Disabled  TRSumVariant=Passthrough  SumFdbkVariant=Disabled  SumVariant=Passthrough_P  TsampFilterVariant=InternalTs  TsampNgainVariant=Passthrough  TsampIntegralVariant=Disabled_SignalSpec
  Saturation : Saturate  UpperLimit=dx_sp_max  LowerLimit=dx_sp_min
  Saturation1 : Saturate  UpperLimit=dz_sp_max  LowerLimit=dz_sp_min
  Sum : Sum  Inputs=|+-
  Sum1 : Sum  Inputs=++|
  Sum2 : Sum  Inputs=|+-
  Sum3 : Sum  Inputs=++|
  k_p : Gain  Gain=kp_x
  k_p1 : Gain  Gain=kp_z
  dX_sp : Outport
  wires:
  Sum/1 -> PID Controller/1, k_p/1
  k_p/1 -> Sum1/2
  PID Controller/1 -> Sum1/1
  X_sp/1 -> Demux/1
  Demux/2 -> [z_sp]
  Demux/1 -> [x_sp]
  X/1 -> Demux1/1
  Demux1/1 -> [x]
  Demux1/2 -> [z]
  [x_sp] -> Sum/1
  [x] -> Sum/2
  Sum2/1 -> PID Controller1/1, k_p1/1
  [z] -> Sum2/2
  [z_sp] -> Sum2/1
  PID Controller1/1 -> Sum3/1
  k_p1/1 -> Sum3/2
  Mux/1 -> dX_sp/1
  Sum1/1 -> Saturation/1
  Sum3/1 -> Saturation1/1
  Saturation1/1 -> Mux/2
  Saturation/1 -> Mux/1

== system linear_flight_controller_payload/PID controllers and Plant/Subsystem1 ==
  X : Inport
  Demux : Demux  Outputs=nx
  theta : Outport
  wires:
  X/1 -> Demux/1
  Demux/3 -> theta/1

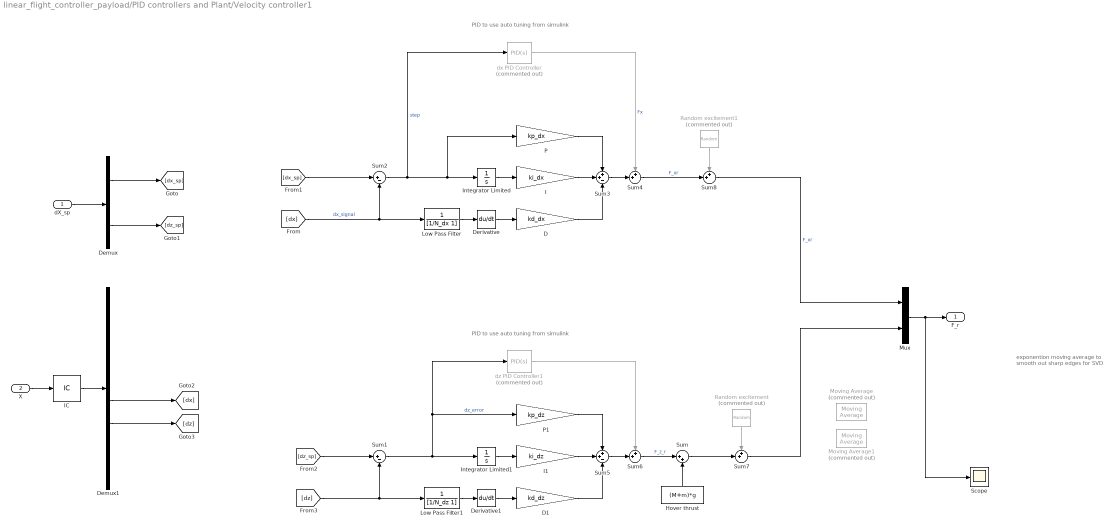
== system linear_flight_controller_payload/PID controllers and Plant/Velocity controller1 ==
  note: exponention moving average
      | to smooth out sharp edges for SVD
  note: PID to use auto tuning from simulink
  note: PID to use auto tuning from simulink
  dX_sp : Inport
  X : Inport  Port=2
  D : Gain  Gain=kd_dx
  D1 : Gain  Gain=kd_dz
  Demux : Demux  Outputs=2
  Demux1 : Demux  Outputs=nx
  Derivative : Derivative
  Derivative1 : Derivative
  Hover thrust : Constant  Value=(M+m)*g
  I : Gain  Gain=ki_dx
  I1 : Gain  Gain=ki_dz
  IC : InitialCondition  Value=x0
  Integrator Limited : Integrator  LimitOutput=on  UpperSaturationLimit=10  LowerSaturationLimit=-10
  Integrator Limited1 : Integrator  LimitOutput=on  UpperSaturationLimit=10  LowerSaturationLimit=-10
  Low Pass Filter : TransferFcn  Denominator=[1/N_dx 1]
  Low Pass Filter1 : TransferFcn  Denominator=[1/N_dz 1]
  Moving Average : dspstat3/Moving Average  Commented=on  Method=Exponential weighting  ForgettingFactorPort=off  SpecifyWindowLength=on  WindowLength=4  ForgettingFactor=lambda  SimulateUsing=Code generation
  Moving Average1 : dspstat3/Moving Average  Commented=on  Method=Exponential weighting  ForgettingFactorPort=off  SpecifyWindowLength=on  WindowLength=4  ForgettingFactor=lambda  SimulateUsing=Code generation
  Mux : Mux  Inputs=2
  P : Gain  Gain=kp_dx
  P1 : Gain  Gain=kp_dz
  Random excitement : RandomNumber  Commented=on  Variance=var_excite  SampleTime=Ts_excite
  Random excitement1 : RandomNumber  Commented=on  Variance=var_excite  Seed=1  SampleTime=Ts_excite
  Scope : Scope
  Sum : Sum  Inputs=|++
  Sum1 : Sum  Inputs=|+-
  Sum2 : Sum  Inputs=|+-
  Sum3 : Sum  Inputs=++-
  Sum{4,6..8} (4 alike) : Sum  Inputs=++|
  Sum5 : Sum  Inputs=++-
  dx PID Controller : simulink/Continuous/PID Controller  Commented=on  Controller=PID  Form=Parallel  TimeDomain=Continuous-time  UseExternalTs=off  SampleTime=-1  IntegratorMethod=Forward Euler  FilterMethod=Forward Euler  ControllerParametersSource=internal  P=kp_dx  I=ki_dx  D=kd_dx  UseFilter=on  N=N_dx  TunerSelectOption=Transfer Function Based (PID Tuner App)  InitialConditionSource=internal  InitialConditionForIntegrator=0  InitialConditionForFilter=0  DifferentiatorICPrevScaledInput=0  ExternalReset=none  TrackingMode=off  Kt=1  LimitOutput=off  UpperSaturationLimit=inf  LowerSaturationLimit=-inf  LinearizeAsGain=on  AntiWindupMode=none  Kb=1  POutMin=[]  POutMax=[]  IOutMin=[]  IOutMax=[]  DOutMin=[]  DOutMax=[]  NOutMin=[]  NOutMax=[]  SumOutMin=[]  SumOutMax=[]  SaturationOutMin=[]  SaturationOutMax=[]  PParamMin=[]  PParamMax=[]  IParamMin=[]  IParamMax=[]  DParamMin=[]  DParamMax=[]  NParamMin=[]  NParamMax=[]  KbParamMin=[]  KbParamMax=[]  KtParamMin=[]  KtParamMax=[]  KbOutMin=[]  KbOutMax=[]  KtOutMin=[]  KtOutMax=[]  IntegratorOutMin=[]  IntegratorOutMax=[]  FilterOutMin=[]  FilterOutMax=[]  SumI1OutMin=[]  SumI1OutMax=[]  SumI2OutMin=[]  SumI2OutMax=[]  SumI3OutMin=[]  SumI3OutMax=[]  SumI4OutMin=[]  SumI4OutMax=[]  SumDOutMin=[]  SumDOutMax=[]  DifferentiatorOutMin=[]  DifferentiatorOutMax=[]  FilterDiffOutCoefMin=[]  FilterDiffOutCoefMax=[]  ReciprocalOutMin=[]  ReciprocalOutMax=[]  SumDenOutMin=[]  SumDenOutMax=[]  SumNumOutMin=[]  SumNumOutMax=[]  DivideOutMin=[]  DivideOutMax=[]  UdiffTsProdOutMin=[]  UdiffTsProdOutMax=[]  NTsProdOutMin=[]  NTsProdOutMax=[]  UintegralTsProdOutMin=[]  UintegralTsProdOutMax=[]  UngainTsProdOutMin=[]  UngainTsProdOutMax=[]  IntegratorContinuousStateAttributes=''  IntegratorStateMustResolveToSignalObject=off  IntegratorRTWStateStorageClass=Auto  FilterContinuousStateAttributes=''  FilterStateMustResolveToSignalObject=off  FilterRTWStateStorageClass=Auto  ParallelPVariant=InternalParameters  IdealPVariant=Disabled  IVariant=InternalParameters  DVariant=InternalParameters  IntegratorVariant=Continuous  SatVariant=Disabled  AWVariant=Passthrough  PCopyVariant=Disabled  TRVariant=Disabled  FdbkBlocksVariant=Forward  IdealPFdbkVariant=Disabled  SatFdbkVariant=Disabled  DerivativeFilterVariant=ContFilter  NVariant=InternalParameters  NCopyVariant=Disabled  FilterICVariant=InternalICsFilter  IntegratorICVariant=InternalICs  ExternalResetVariant=Disabled  TRSumVariant=Passthrough  SumFdbkVariant=Disabled  SumVariant=Sum_PID  TsampFilterVariant=InternalTs  TsampNgainVariant=Passthrough  TsampIntegralVariant=Passthrough
  dz PID Controller1 : simulink/Continuous/PID Controller  Commented=on  Controller=PID  Form=Parallel  TimeDomain=Continuous-time  UseExternalTs=off  SampleTime=-1  IntegratorMethod=Forward Euler  FilterMethod=Forward Euler  ControllerParametersSource=internal  P=kp_dz  I=ki_dz  D=kd_dz  UseFilter=on  N=N_dz  TunerSelectOption=Transfer Function Based (PID Tuner App)  InitialConditionSource=internal  InitialConditionForIntegrator=0  InitialConditionForFilter=0  DifferentiatorICPrevScaledInput=0  ExternalReset=none  TrackingMode=off  Kt=1  LimitOutput=off  UpperSaturationLimit=inf  LowerSaturationLimit=-inf  LinearizeAsGain=on  AntiWindupMode=none  Kb=1  POutMin=[]  POutMax=[]  IOutMin=[]  IOutMax=[]  DOutMin=[]  DOutMax=[]  NOutMin=[]  NOutMax=[]  SumOutMin=[]  SumOutMax=[]  SaturationOutMin=[]  SaturationOutMax=[]  PParamMin=[]  PParamMax=[]  IParamMin=[]  IParamMax=[]  DParamMin=[]  DParamMax=[]  NParamMin=[]  NParamMax=[]  KbParamMin=[]  KbParamMax=[]  KtParamMin=[]  KtParamMax=[]  KbOutMin=[]  KbOutMax=[]  KtOutMin=[]  KtOutMax=[]  IntegratorOutMin=[]  IntegratorOutMax=[]  FilterOutMin=[]  FilterOutMax=[]  SumI1OutMin=[]  SumI1OutMax=[]  SumI2OutMin=[]  SumI2OutMax=[]  SumI3OutMin=[]  SumI3OutMax=[]  SumI4OutMin=[]  SumI4OutMax=[]  SumDOutMin=[]  SumDOutMax=[]  DifferentiatorOutMin=[]  DifferentiatorOutMax=[]  FilterDiffOutCoefMin=[]  FilterDiffOutCoefMax=[]  ReciprocalOutMin=[]  ReciprocalOutMax=[]  SumDenOutMin=[]  SumDenOutMax=[]  SumNumOutMin=[]  SumNumOutMax=[]  DivideOutMin=[]  DivideOutMax=[]  UdiffTsProdOutMin=[]  UdiffTsProdOutMax=[]  NTsProdOutMin=[]  NTsProdOutMax=[]  UintegralTsProdOutMin=[]  UintegralTsProdOutMax=[]  UngainTsProdOutMin=[]  UngainTsProdOutMax=[]  IntegratorContinuousStateAttributes=''  IntegratorStateMustResolveToSignalObject=off  IntegratorRTWStateStorageClass=Auto  FilterContinuousStateAttributes=''  FilterStateMustResolveToSignalObject=off  FilterRTWStateStorageClass=Auto  ParallelPVariant=InternalParameters  IdealPVariant=Disabled  IVariant=InternalParameters  DVariant=InternalParameters  IntegratorVariant=Continuous  SatVariant=Disabled  AWVariant=Passthrough  PCopyVariant=Disabled  TRVariant=Disabled  FdbkBlocksVariant=Forward  IdealPFdbkVariant=Disabled  SatFdbkVariant=Disabled  DerivativeFilterVariant=ContFilter  NVariant=InternalParameters  NCopyVariant=Disabled  FilterICVariant=InternalICsFilter  IntegratorICVariant=InternalICs  ExternalResetVariant=Disabled  TRSumVariant=Passthrough  SumFdbkVariant=Disabled  SumVariant=Sum_PID  TsampFilterVariant=InternalTs  TsampNgainVariant=Passthrough  TsampIntegralVariant=Passthrough
  F_r : Outport
  wires:
  Derivative/1 -> D/1
  Sum3/1 -> Sum4/2
  Sum2/1 -> dx PID Controller/1, P/1, Integrator Limited/1  "step"
  I/1 -> Sum3/2
  Integrator Limited/1 -> I/1
  dx PID Controller/1 -> Sum4/1  "Fx"
  P/1 -> Sum3/1
  Low Pass Filter/1 -> Derivative/1
  D/1 -> Sum3/3
  P1/1 -> Sum5/1
  Integrator Limited1/1 -> I1/1
  dz PID Controller1/1 -> Sum6/1
  I1/1 -> Sum5/2
  Sum1/1 -> P1/1, dz PID Controller1/1, Integrator Limited1/1  "dz_error"
  Sum5/1 -> Sum6/2
  Low Pass Filter1/1 -> Derivative1/1
  Derivative1/1 -> D1/1
  D1/1 -> Sum5/3
  dX_sp/1 -> Demux/1
  [dx] -> Sum2/2, Low Pass Filter/1  "dx_signal"
  [dx_sp] -> Sum2/1
  Demux/1 -> [dx_sp]
  Demux/2 -> [dz_sp]
  [dz] -> Sum1/2, Low Pass Filter1/1
  [dz_sp] -> Sum1/1
  Demux1/5 -> [dx]
  Demux1/6 -> [dz]
  Sum6/1 -> Sum/1  "F_z_r"
  Hover thrust/1 -> Sum/2
  IC/1 -> Demux1/1
  X/1 -> IC/1
  Sum8/1 -> Mux/1  "F_xr"
  Sum7/1 -> Mux/2
  Mux/1 -> Scope/1, F_r/1
  Random excitement/1 -> Sum7/1
  Sum/1 -> Sum7/2
  Random excitement1/1 -> Sum8/1
  Sum4/1 -> Sum8/2  "F_xr"

== system linear_flight_controller_payload/state space WITHOUT payload1/Angle controller1 ==
  theta_sp : Inport
  X : Inport  Port=2
  Demux1 : Demux  Outputs=6
  Gain : Gain  Gain=kp_theta
  PID Controller : simulink/Continuous/PID Controller  Commented=on  Controller=P  Form=Parallel  TimeDomain=Continuous-time  UseExternalTs=off  SampleTime=-1  IntegratorMethod=Forward Euler  FilterMethod=Forward Euler  ControllerParametersSource=internal  P=kp_theta  I=1  D=0  UseFilter=on  N=100  TunerSelectOption=Transfer Function Based (PID Tuner App)  InitialConditionSource=internal  InitialConditionForIntegrator=0  InitialConditionForFilter=0  DifferentiatorICPrevScaledInput=0  ExternalReset=none  TrackingMode=off  Kt=1  LimitOutput=off  UpperSaturationLimit=inf  LowerSaturationLimit=-inf  LinearizeAsGain=on  AntiWindupMode=none  Kb=1  POutMin=[]  POutMax=[]  IOutMin=[]  IOutMax=[]  DOutMin=[]  DOutMax=[]  NOutMin=[]  NOutMax=[]  SumOutMin=[]  SumOutMax=[]  SaturationOutMin=[]  SaturationOutMax=[]  PParamMin=[]  PParamMax=[]  IParamMin=[]  IParamMax=[]  DParamMin=[]  DParamMax=[]  NParamMin=[]  NParamMax=[]  KbParamMin=[]  KbParamMax=[]  KtParamMin=[]  KtParamMax=[]  KbOutMin=[]  KbOutMax=[]  KtOutMin=[]  KtOutMax=[]  IntegratorOutMin=[]  IntegratorOutMax=[]  FilterOutMin=[]  FilterOutMax=[]  SumI1OutMin=[]  SumI1OutMax=[]  SumI2OutMin=[]  SumI2OutMax=[]  SumI3OutMin=[]  SumI3OutMax=[]  SumI4OutMin=[]  SumI4OutMax=[]  SumDOutMin=[]  SumDOutMax=[]  DifferentiatorOutMin=[]  DifferentiatorOutMax=[]  FilterDiffOutCoefMin=[]  FilterDiffOutCoefMax=[]  ReciprocalOutMin=[]  ReciprocalOutMax=[]  SumDenOutMin=[]  SumDenOutMax=[]  SumNumOutMin=[]  SumNumOutMax=[]  DivideOutMin=[]  DivideOutMax=[]  UdiffTsProdOutMin=[]  UdiffTsProdOutMax=[]  NTsProdOutMin=[]  NTsProdOutMax=[]  UintegralTsProdOutMin=[]  UintegralTsProdOutMax=[]  UngainTsProdOutMin=[]  UngainTsProdOutMax=[]  IntegratorContinuousStateAttributes=''  IntegratorStateMustResolveToSignalObject=off  IntegratorRTWStateStorageClass=Auto  FilterContinuousStateAttributes=''  FilterStateMustResolveToSignalObject=off  FilterRTWStateStorageClass=Auto  ParallelPVariant=InternalParameters  IdealPVariant=Disabled  IVariant=Disabled  DVariant=Disabled  IntegratorVariant=Disabled  SatVariant=Disabled  AWVariant=Disabled  PCopyVariant=Disabled  TRVariant=Disabled  FdbkBlocksVariant=Forward  IdealPFdbkVariant=Disabled  SatFdbkVariant=Disabled  DerivativeFilterVariant=Disabled  NVariant=Disabled  NCopyVariant=Disabled_SignalSpec  FilterICVariant=Disabled  IntegratorICVariant=Disabled  ExternalResetVariant=Disabled  TRSumVariant=Passthrough  SumFdbkVariant=Disabled  SumVariant=Passthrough_P  TsampFilterVariant=InternalTs  TsampNgainVariant=Passthrough  TsampIntegralVariant=Disabled_SignalSpec
  Sum : Sum  Inputs=++|
  Sum1 : Sum  Inputs=|+-
  limit : Saturate  UpperLimit=dtheta_sp_max  LowerLimit=dtheta_sp_min
  dtheta_sp : Outport
  wires:
  Sum1/1 -> PID Controller/1, Gain/1  "theta_error"
  theta_sp/1 -> Sum1/1
  PID Controller/1 -> Sum/1
  Gain/1 -> Sum/2
  X/1 -> Demux1/1
  Demux1/3 -> Sum1/2
  Sum/1 -> limit/1
  limit/1 -> dtheta_sp/1
